simulink model "BladeRF_rx_sin"  (R2023a)
settings: Solver=FixedStepDiscrete  StartTime=0.0  StopTime=inf  RelTol=1e-3
undefined symbols (not defined in the file or in its folder): physconst
libraries: phaseddoalib x2, dspspect3 x1, dspsrcs4 x1, dspmathops x1
settings Model: SimulationMode=accelerator  Creator=memre  LastModifiedBy=memre
settings DebuggingCC: ParameterPrecisionLossMsg=none

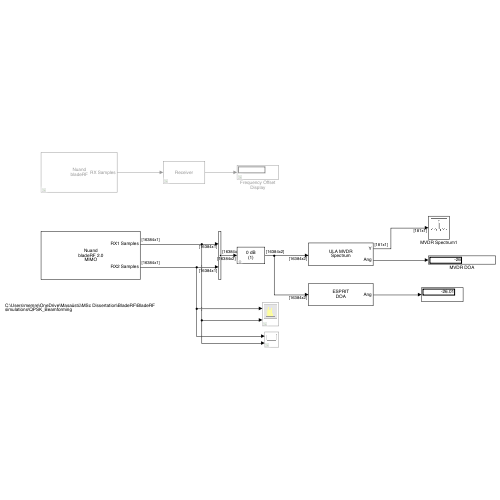
[thumbnail: Simulink's stored preview of the top-level diagram]
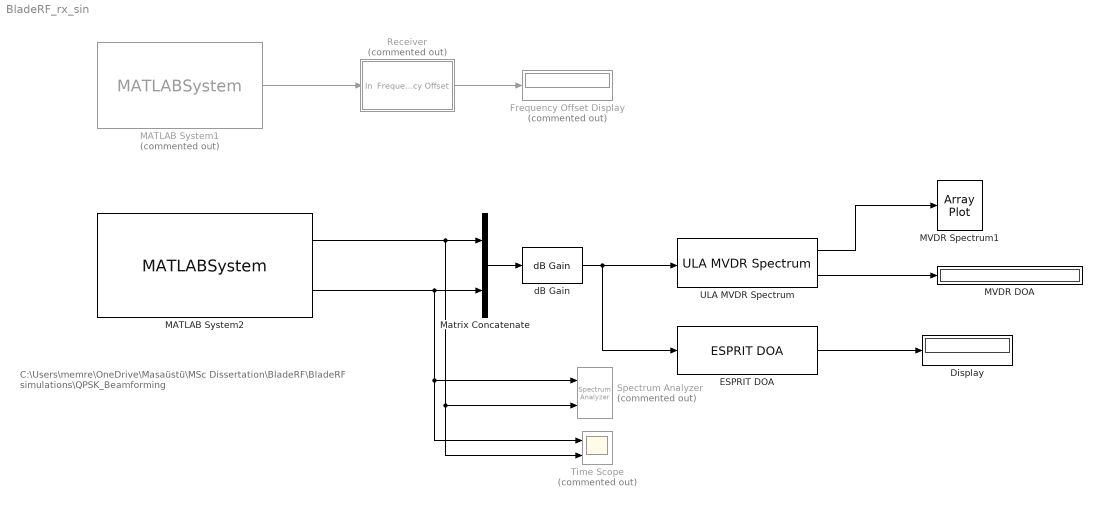
== system BladeRF_rx_sin ==
  note: C:\Users\memre\OneDrive\Masaüstü\MSc Dissertation\BladeRF\BladeRF simulations\QPSK_Beamforming
  Display : Display
  ESPRIT DOA : phaseddoalib/ESPRIT DOA  PropagationSpeed=physconst( 'LightSpeed' )  OperatingFrequency=915e6  NumSignalsSource=Property  NumSignalsMethod=AIC  NumSignals=1  SpatialSmoothing=0  Method=TLS  ForwardBackwardAveraging=off  RowWeighting=1  SimulateUsing=Interpreted execution  SensorArray=Rx_Antennas
  Frequency Offset Display : Display  Commented=on
  MATLAB System1 : MATLABSystem  Commented=on  System=bladeRF_Simulink  device_string=*:instance=0  loopback_mode=None  xb200=off  SimulateUsing=Interpreted execution  enable_rx=on  enable_overrun=off  rx_frequency=2.4e9 - 1746  rx_samplerate=1e6  rx_bandwidth=1.5  rx_gain=50  enable_rx_biastee=off  rx_agc=SLOW  rx_num_buffers=256  rx_num_transfers=8  rx_buf_size=16384  rx_timeout_ms=3500  rx_step_size=16384  enable_tx=off  enable_underrun=off  tx_frequency=2.4e9  tx_samplerate=1e6  tx_bandwidth=1.5  tx_gain=70  enable_tx_biastee=off  tx_num_buffers=256  tx_num_transfers=8  tx_buf_size=16384  tx_timeout_ms=3500  tx_step_size=16384  verbosity=Info
      mask Type: bladeRF_Simulink
      mask Display:
      | disp(['Nuand' char(10) 'bladeRF']);
      | port_label('output',1,'RX Samples');
  MATLAB System2 : MATLABSystem  System=bladeRF_MIMO_Simulink  device_string=*:instance=0  loopback_mode=None  xb200=off  SimulateUsing=Interpreted execution  enable_rx=on  enable_overrun=off  rx_frequency=915e6  rx_samplerate=1e6  rx_bandwidth=1.5  rx_gain=70  enable_rx_biastee=off  rx_agc=MANUAL  rx_num_buffers=16*2  rx_num_transfers=8  rx_buf_size=16384*2  rx_timeout_ms=5000  rx_step_size=16384  enable_rx2=on  rx2_frequency=915e6  rx2_samplerate=1e6  rx2_bandwidth=1.5  rx2_gain=70  enable_rx2_biastee=off  rx2_agc=MANUAL  enable_tx=off  enable_underrun=off  tx_frequency=915e6  tx_samplerate=3e6  tx_bandwidth=1.5  tx_gain=60  enable_tx_biastee=off  tx_num_buffers=64  tx_num_transfers=16  tx_buf_size=16384  tx_timeout_ms=5000  tx_step_size=16384  enable_tx2=off  tx2_frequency=915e6  tx2_samplerate=3e6  tx2_bandwidth=1.5  tx2_gain=60  enable_tx2_biastee=off  verbosity=Info
      mask Type: bladeRF_MIMO_Simulink
      mask Display:
      | disp(['Nuand' char(10) 'bladeRF 2.0' char(10) 'MIMO']);
      | port_label('output',1,'RX1 Samples');
      | port_label('output',2,'RX2 Samples');
  MVDR DOA : Display
  MVDR Spectrum1 : ArrayPlot  WindowPosition=[135.000000,250.000000,1050.000000,666.000000,]  ScopeFrameLocation=window  XOffset=10  PlotType=Line  AxesScaling=Manual  Title=MVDR Spectrum  XLabel=Angle (degrees)  YLabel=Magnitude  YLimits=[-1,10]  ShowLegend=on  DefaultConfigurationName=dsp.scopes.ArrayPlotBlockSpecification
  Matrix Concatenate : Concatenate  Mode=Multidimensional array  ConcatenateDimension=2
  Receiver : Subsystem  Commented=on
      mask Display: disp('Receiver')
  Spectrum Analyzer : SpectrumAnalyzer  Commented=on  NumInputPorts=2  WindowPosition=[386.000000,244.000000,807.000000,547.000000,]  ScopeFrameLocation=window  SpectrumType=Power density  Method=Welch  SampleRate=100000  AxesScaling=Manual  Span=200000  StartFrequency=-100000  StopFrequency=100000  FFTLengthSource=Property  FFTLength=8192  WindowLength=4096  AveragingMethod=Running  SpectralAverages=10  SpectrumUnits=dBW/Hz  YLabel=Magnitude-squared, dB  YLimits=[-123.49488151760544,-15.327792116023211]  ShowLegend=on
  Time Scope : Scope  Commented=on  NumInputPorts=2
  ULA MVDR Spectrum : phaseddoalib/ULA MVDR Spectrum  PropagationSpeed=physconst( 'LightSpeed' )  OperatingFrequency=915e6  NumPhaseShifterBits=0  ForwardBackwardAveraging=off  SpatialSmoothing=0  ScanAngles=-90:90  DOAOutputPort=on  NumSignals=1  SimulateUsing=Interpreted execution  SensorArray=Rx_Antennas
  dB Gain : dspmathops/dB Gain  dB=0  intype=Amplitude
  wires:
  MATLAB System1/1 -> Receiver/1(In)
  Receiver/1(Frequency Offset) -> Frequency Offset Display/1
  MATLAB System2/2 -> Spectrum Analyzer/1, Time Scope/1, Matrix Concatenate/2
  MATLAB System2/1 -> Time Scope/2, Spectrum Analyzer/2, Matrix Concatenate/1
  ULA MVDR Spectrum/1 -> MVDR Spectrum1/1
  ULA MVDR Spectrum/2 -> MVDR DOA/1
  Matrix Concatenate/1 -> dB Gain/1
  dB Gain/1 -> ESPRIT DOA/1, ULA MVDR Spectrum/1
  ESPRIT DOA/1 -> Display/1

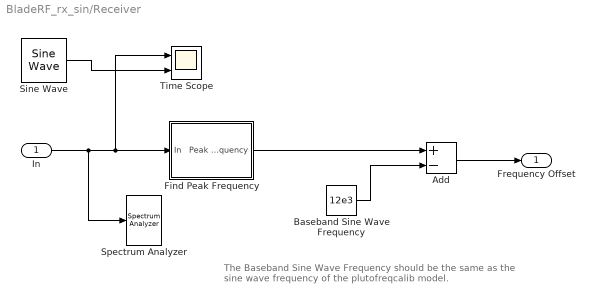
== system BladeRF_rx_sin/Receiver ==
  note: The Baseband Sine Wave Frequency should be the same as
      | the sine wave frequency of the plutofreqcalib model.
  In : Inport
  Add : Sum  Inputs=+-
  Baseband Sine Wave Frequency : Constant  Value=12e3
  Find Peak Frequency : Subsystem
      mask Display: disp('Find Peak\nFrequency')
  Sine Wave : dspsrcs4/Sine Wave  Amplitude=1  Frequency=12000  Phase=0  SampleMode=Discrete  OutComplex=Complex  CompMethod=Trigonometric fcn  TableSize=Speed  SampleTime=1/1e6  SamplesPerFrame=16384  ResetState=Restart at time zero  OutputFrames=off  dataType=double  wordLen=16  udDataType=sfix(16)  fracBitsMode=Best precision  numFracBits=15  OutDataTypeStr=double  LastOutDataTypeStr=double
  Spectrum Analyzer : SpectrumAnalyzer  WindowPosition=[386.000000,244.000000,807.000000,467.000000,]  ScopeFrameLocation=window  SpectrumType=Power density  Method=Welch  SampleRate=100000  AxesScaling=Manual  Span=200000  StartFrequency=-100000  StopFrequency=100000  FFTLengthSource=Property  FFTLength=8192  WindowLength=4096  AveragingMethod=Running  SpectralAverages=10  SpectrumUnits=dBW/Hz  YLabel=Magnitude-squared, dB  YLimits=[-123.49488151760544,-15.327792116023211]
  Time Scope : Scope  NumInputPorts=2
  Frequency Offset : Outport  VectorParamsAs1DForOutWhenUnconnected=off
  wires:
  Find Peak Frequency/1(Peak Frequency) -> Add/1
  Baseband Sine Wave Frequency/1 -> Add/2
  Add/1 -> Frequency Offset/1
  In/1 -> Spectrum Analyzer/1, Time Scope/1, Find Peak Frequency/1(In)
  Sine Wave/1 -> Time Scope/2

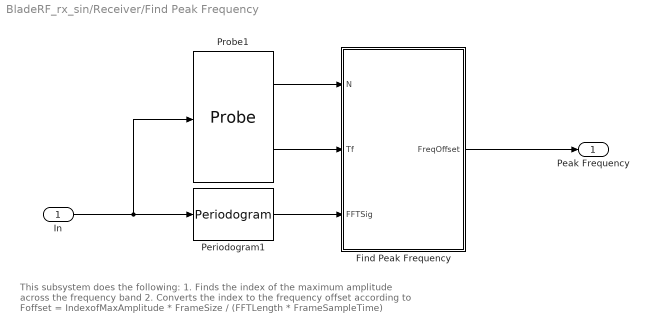
== system BladeRF_rx_sin/Receiver/Find Peak Frequency ==
  note: This subsystem does the following:
      | 1.  Finds the index of the maximum amplitude across the frequency band
      | 2.  Converts the index to the frequency offset according to
      | Foffset = IndexofMaxAmplitude * FrameSize / (FFTLength * FrameSampleTime)
  In : Inport
  Find Peak Frequency : MATLAB Function  TreatAsAtomicUnit=on
  Periodogram1 : dspspect3/Periodogram  measurement=Power spectral density  wintype=Hamming  Rs=50  beta=5  winsamp=Symmetric  FFTImplementation=Auto  inheritFFT=off  fftsize=2048  navg=2  inheritTs=on  Ts=1
  Probe1 : Probe  ProbeComplexSignal=off
  Peak Frequency : Outport  VectorParamsAs1DForOutWhenUnconnected=off
  wires:
  Periodogram1/1 -> Find Peak Frequency/3(FFTSig)
  Probe1/1 -> Find Peak Frequency/1(N)
  Probe1/2 -> Find Peak Frequency/2(Tf)
  Find Peak Frequency/1(FreqOffset) -> Peak Frequency/1
  In/1 -> Periodogram1/1, Probe1/1

== matlab function BladeRF_rx_sin/Receiver/Find Peak Frequency/Find Peak Frequency ==
  data: N input; FreqOffset output; Tf input; FFTSig input
function FreqOffset  = findpeakfreq(N, Tf, FFTSig)
% Find peak frequency
% N - frame size
% Tf - frame sample time
% FFTSig - result of FFT

%#codegen

FFTSize = length(FFTSig);
FFTSig = fftshift(FFTSig);
[~, maxIdx] = max(FFTSig); % Find index of max magnitude
OffsetIdx = maxIdx-1-FFTSize/2; % Convert to index symmetric with 0
Ts = Tf(1)/N; % Sample time
delta_f = 1/Ts/FFTSize; % Frequency resolution of FFT
FreqOffset = OffsetIdx*delta_f;% Map offset index back to frequency
